simulink model "third_1"  (R2025a)
settings: Solver=VariableStepAuto  StartTime=0.0  StopTime=3  RelTol=1e-3
libraries: simulink x1
settings Model: Creator=28097  LastModifiedBy=28097

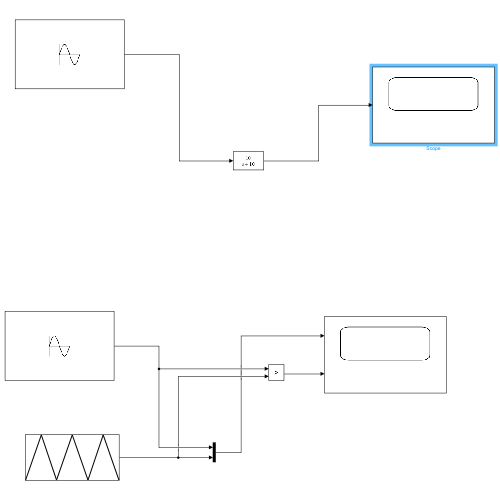
[thumbnail: Simulink's stored preview of the top-level diagram]
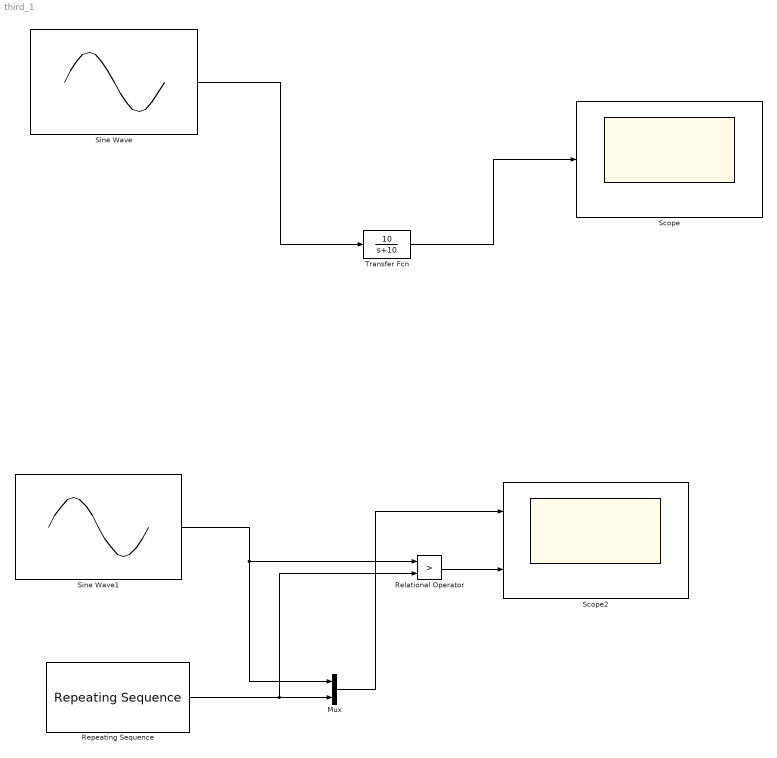
== system third_1 ==
  Mux : Mux  Inputs=2
  Relational Operator : RelationalOperator  Operator=>  OutDataTypeStr=boolean  RndMeth=Simplest  InputSameDT=off
  Repeating Sequence : simulink/Sources/Repeating Sequence  rep_seq_t=[0 0.025 0.05]  rep_seq_y=[-1 1 -1]
  Scope : Scope
      settings: ActiveDisplayYMinimum=-5.5216379231475265  ActiveDisplayYMaximum=4.9178904526875709
  Scope2 : Scope  NumInputPorts=2
      settings: ActiveDisplayYMinimum=-4.9180676675432231  ActiveDisplayYMaximum=3.4285645775751856  DataLoggingVariableName=ScopeData2
  Sine Wave : Sin  Frequency=2*pi*1  SampleTime=0
  Sine Wave1 : Sin  Amplitude=0.8  Frequency=2*pi*1  SampleTime=0
  Transfer Fcn : TransferFcn  Numerator=[10]  Denominator=[1 10]
  wires:
  Transfer Fcn/1 -> Scope/1
  Sine Wave1/1 -> Relational Operator/1, Mux/1
  Repeating Sequence/1 -> Relational Operator/2, Mux/2
  Mux/1 -> Scope2/1
  Relational Operator/1 -> Scope2/2
  Sine Wave/1 -> Transfer Fcn/1
